simulink model "CM012A_FordT3McuCfg"  (R2013b)
settings: Solver=FixedStepDiscrete  SolverMode=SingleTasking  StartTime=0.0  StopTime=2  FixedStep=0.00005  RelTol=1e-3
values from neighbouring files (symbols this model uses):
  BATTVLTGSCAGFAC_ULS_F32 = DataDict.Constant    [CM012A_FordT3McuCfg_DataDict.m]
  BATTVLTGSWD1SCAGFAC_ULS_F32 = DataDict.Constant    [CM012A_FordT3McuCfg_DataDict.m]
  CHRGPMPDIAGSCAGFAC_ULS_F32 = DataDict.Constant    [CM012A_FordT3McuCfg_DataDict.m]
  MOTAG2MEAS_ECU1OFFS_MOTREV_F32 = DataDict.Constant    [CM012A_FordT3McuCfg_DataDict.m]
  MOTAG2MEAS_ECU2OFFS_MOTREV_F32 = DataDict.Constant    [CM012A_FordT3McuCfg_DataDict.m]
  PWRDISCNCTSWTDIAGSCAGFAC_ULS_F32 = DataDict.Constant    [CM012A_FordT3McuCfg_DataDict.m]
undefined symbols (not defined in the file or in its folder): HwAgSnsrTyp1, sigbuilder_block
libraries: CM012A_FordT3McuCfg_ModelLibrary x114, simulink x37, NxtrLim x34
(part 3 of 4)

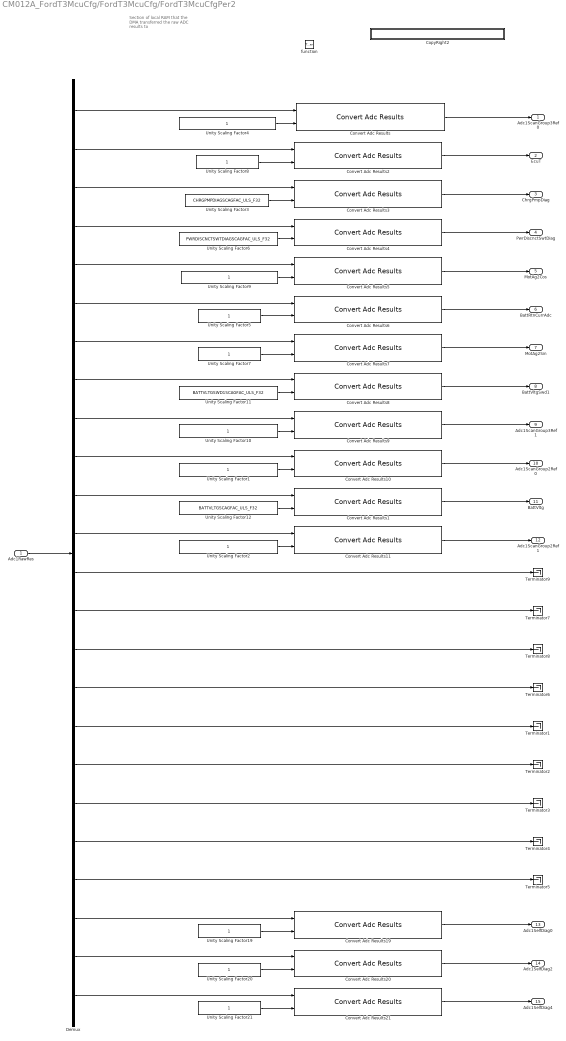
== system CM012A_FordT3McuCfg/FordT3McuCfg/FordT3McuCfgPer2 ==
  note: Section of local RAM that the
      | DMA transferred the raw
      | ADC results to
  Adc1RawRes : Inport
  function : TriggerPort  TriggerType=function-call
  Convert Adc Results{,9..11,19..21} (7 alike) : CM012A_FordT3McuCfg_ModelLibrary/Convert Adc Results
  Convert Adc Results1 : CM012A_FordT3McuCfg_ModelLibrary/Convert Adc Results  RequirementInfo="{'linktype_rmi_doors' '00016ba8 (/ESG Group/FDD Module Requirements/EA4 Specific/CM012A_FordT3McuCfg)' '#CM012A_185' 'true' 'REQ:  CM012A_185' '' } %GIDa_5e3dfbd3_0aa2_4a0d_bf3e_86a251f38de3"
  Convert Adc Results2 : CM012A_FordT3McuCfg_ModelLibrary/Convert Adc Results  RequirementInfo="{'linktype_rmi_doors' '00016ba8 (/ESG Group/FDD Module Requirements/EA4 Specific/CM012A_FordT3McuCfg)' '#CM012A_178' 'true' 'REQ:  CM012A_178' '' } %GIDa_a26960ee_7e00_4846_9982_291370be49c9"
  Convert Adc Results3 : CM012A_FordT3McuCfg_ModelLibrary/Convert Adc Results  RequirementInfo="{'linktype_rmi_doors' '00016ba8 (/ESG Group/FDD Module Requirements/EA4 Specific/CM012A_FordT3McuCfg)' '#CM012A_179' 'true' 'REQ:  CM012A_179' '' } %GIDa_a9d1aa2c_659d_4b57_940c_077b57984895"
  Convert Adc Results4 : CM012A_FordT3McuCfg_ModelLibrary/Convert Adc Results  RequirementInfo="{'linktype_rmi_doors' '00016ba8 (/ESG Group/FDD Module Requirements/EA4 Specific/CM012A_FordT3McuCfg)' '#CM012A_180' 'true' 'REQ:  CM012A_180' '' } %GIDa_849e543f_3e98_4047_be72_b68ed64419df"
  Convert Adc Results5 : CM012A_FordT3McuCfg_ModelLibrary/Convert Adc Results  RequirementInfo="{'linktype_rmi_doors' '00016ba8 (/ESG Group/FDD Module Requirements/EA4 Specific/CM012A_FordT3McuCfg)' '#CM012A_181' 'true' 'REQ:  CM012A_181' '' } %GIDa_b9fd61a2_c26d_490b_9ec2_e1953f6cec27"
  Convert Adc Results6 : CM012A_FordT3McuCfg_ModelLibrary/Convert Adc Results  RequirementInfo="{'linktype_rmi_doors' '00016ba8 (/ESG Group/FDD Module Requirements/EA4 Specific/CM012A_FordT3McuCfg)' '#CM012A_182' 'true' 'REQ:  CM012A_182' '' } %GIDa_1805e95d_a947_4975_b3f2_aa5b017a8660"
  Convert Adc Results7 : CM012A_FordT3McuCfg_ModelLibrary/Convert Adc Results  RequirementInfo="{'linktype_rmi_doors' '00016ba8 (/ESG Group/FDD Module Requirements/EA4 Specific/CM012A_FordT3McuCfg)' '#CM012A_183' 'true' 'REQ:  CM012A_183' '' } %GIDa_b0f2763e_6efc_4366_bdd2_7a7ad43f2cd5"
  Convert Adc Results8 : CM012A_FordT3McuCfg_ModelLibrary/Convert Adc Results  RequirementInfo="{'linktype_rmi_doors' '00016ba8 (/ESG Group/FDD Module Requirements/EA4 Specific/CM012A_FordT3McuCfg)' '#CM012A_184' 'true' 'REQ:  CM012A_184' '' } %GIDa_a85505f7_8cc5_414b_b13e_a958c65078c9"
  CopyRight2 : Subsystem  Description=|  mask(Copyright Information){none=on}
      | Copyright info block.                                               
      |                                                                     
      | Place copyright information at the top of every subsystem in design.
      mask prompts: none "No parameters"
      mask help: Place copyright information at the top of every subsystem in design.
      mask Display:
      | NxtrConf = 'Nexteer Confidential';
      | 
      | sys = bdroot; %handle for the current model ("system")
      | first = get_param(sys,'Created');
      | first = first(end-3:end);  %year is last four digits
      | 
      | last = get_param(sys,'LastModifiedDate');
      | if isempty(last)
      |     last = datestr(now,'yyyy');
      | else
      |     last = last(end-3:end);
      | end
      | 
      | if strcmp(first,last)
      |     fprintf('%s -- Copyright %s Nexteer',NxtrConf,first)
      | else
      |     fprintf('%s -- %s%s- %s Nexteer',NxtrConf,char(169),first,last)
      | end
  Demux : Demux  Outputs=24
  Terminator{1..9} (9 alike) : Terminator
  Unity Scaling Factor{1..2,4..5,7..10,19..21} (11 alike) : Constant  OutDataTypeStr=single
  Unity Scaling Factor11 : Constant  RequirementInfo="{'linktype_rmi_doors' '00016ba8 (/ESG Group/FDD Module Requirements/EA4 Specific/CM012A_FordT3McuCfg)' '#CM012A_184' 'true' 'REQ:  CM012A_184' '' } %GIDa_4557c3db_2e6a_4677_b8e3_15478f0550e6"  Value=BATTVLTGSWD1SCAGFAC_ULS_F32
  Unity Scaling Factor12 : Constant  RequirementInfo="{'linktype_rmi_doors' '00016ba8 (/ESG Group/FDD Module Requirements/EA4 Specific/CM012A_FordT3McuCfg)' '#CM012A_185' 'true' 'REQ:  CM012A_185' '' } %GIDa_1deb9cd3_1e38_4031_b7c6_d1408aef7916"  Value=BATTVLTGSCAGFAC_ULS_F32
  Unity Scaling Factor3 : Constant  RequirementInfo="{'linktype_rmi_doors' '00016ba8 (/ESG Group/FDD Module Requirements/EA4 Specific/CM012A_FordT3McuCfg)' '#CM012A_179' 'true' 'REQ:  CM012A_179' '' } %GIDa_de87164e_670f_496e_a314_697b1553e9fe"  Value=CHRGPMPDIAGSCAGFAC_ULS_F32
  Unity Scaling Factor6 : Constant  RequirementInfo="{'linktype_rmi_doors' '00016ba8 (/ESG Group/FDD Module Requirements/EA4 Specific/CM012A_FordT3McuCfg)' '#CM012A_180' 'true' 'REQ:  CM012A_180' '' } %GIDa_80971ee9_65a5_459a_87c3_3a33b74619be"  Value=PWRDISCNCTSWTDIAGSCAGFAC_ULS_F32
  Adc1ScanGroup3Ref0 : Outport
  EcuT : Outport  Port=2
  ChrgPmpDiag : Outport  Port=3
  PwrDiscnctSwtDiag : Outport  Port=4
  MotAg2Cos : Outport  Port=5
  BattRtnCurrAdc : Outport  Port=6
  MotAg2Sin : Outport  Port=7
  BattVltgSwd1 : Outport  Port=8
  Adc1ScanGroup3Ref1 : Outport  Port=9
  Adc1ScanGroup2Ref0 : Outport  Port=10
  BattVltg : Outport  Port=11
  Adc1ScanGroup2Ref1 : Outport  Port=12
  Adc1SelfDiag0 : Outport  Port=13
  Adc1SelfDiag2 : Outport  Port=14
  Adc1SelfDiag4 : Outport  Port=15
  wires:
  Adc1RawRes/1 -> Demux/1
  Demux/1 -> Convert Adc Results/1
  Unity Scaling Factor4/1 -> Convert Adc Results/2
  Convert Adc Results/1 -> Adc1ScanGroup3Ref0/1
  Demux/4 -> Convert Adc Results4/1
  Unity Scaling Factor3/1 -> Convert Adc Results3/2
  Demux/3 -> Convert Adc Results3/1
  Unity Scaling Factor8/1 -> Convert Adc Results2/2
  Demux/2 -> Convert Adc Results2/1
  Unity Scaling Factor6/1 -> Convert Adc Results4/2
  Demux/9 -> Convert Adc Results9/1
  Unity Scaling Factor11/1 -> Convert Adc Results8/2
  Demux/8 -> Convert Adc Results8/1
  Unity Scaling Factor7/1 -> Convert Adc Results7/2
  Demux/7 -> Convert Adc Results7/1
  Unity Scaling Factor5/1 -> Convert Adc Results6/2
  Demux/6 -> Convert Adc Results6/1
  Demux/5 -> Convert Adc Results5/1
  Unity Scaling Factor9/1 -> Convert Adc Results5/2
  Unity Scaling Factor10/1 -> Convert Adc Results9/2
  Convert Adc Results2/1 -> EcuT/1
  Convert Adc Results3/1 -> ChrgPmpDiag/1
  Convert Adc Results4/1 -> PwrDiscnctSwtDiag/1
  Convert Adc Results5/1 -> MotAg2Cos/1
  Convert Adc Results6/1 -> BattRtnCurrAdc/1
  Demux/10 -> Convert Adc Results10/1
  Unity Scaling Factor1/1 -> Convert Adc Results10/2
  Convert Adc Results7/1 -> MotAg2Sin/1
  Convert Adc Results8/1 -> BattVltgSwd1/1
  Convert Adc Results9/1 -> Adc1ScanGroup3Ref1/1
  Convert Adc Results10/1 -> Adc1ScanGroup2Ref0/1
  Unity Scaling Factor12/1 -> Convert Adc Results1/2
  Demux/11 -> Convert Adc Results1/1
  Convert Adc Results1/1 -> BattVltg/1
  Demux/17 -> Terminator1/1
  Demux/18 -> Terminator2/1
  Demux/19 -> Terminator3/1
  Demux/20 -> Terminator4/1
  Demux/21 -> Terminator5/1
  Unity Scaling Factor21/1 -> Convert Adc Results21/2
  Demux/24 -> Convert Adc Results21/1
  Unity Scaling Factor20/1 -> Convert Adc Results20/2
  Demux/23 -> Convert Adc Results20/1
  Unity Scaling Factor19/1 -> Convert Adc Results19/2
  Demux/22 -> Convert Adc Results19/1
  Demux/12 -> Convert Adc Results11/1
  Unity Scaling Factor2/1 -> Convert Adc Results11/2
  Demux/16 -> Terminator6/1
  Demux/14 -> Terminator7/1
  Demux/15 -> Terminator8/1
  Demux/13 -> Terminator9/1
  Convert Adc Results11/1 -> Adc1ScanGroup2Ref1/1
  Convert Adc Results20/1 -> Adc1SelfDiag2/1
  Convert Adc Results19/1 -> Adc1SelfDiag0/1
  Convert Adc Results21/1 -> Adc1SelfDiag4/1

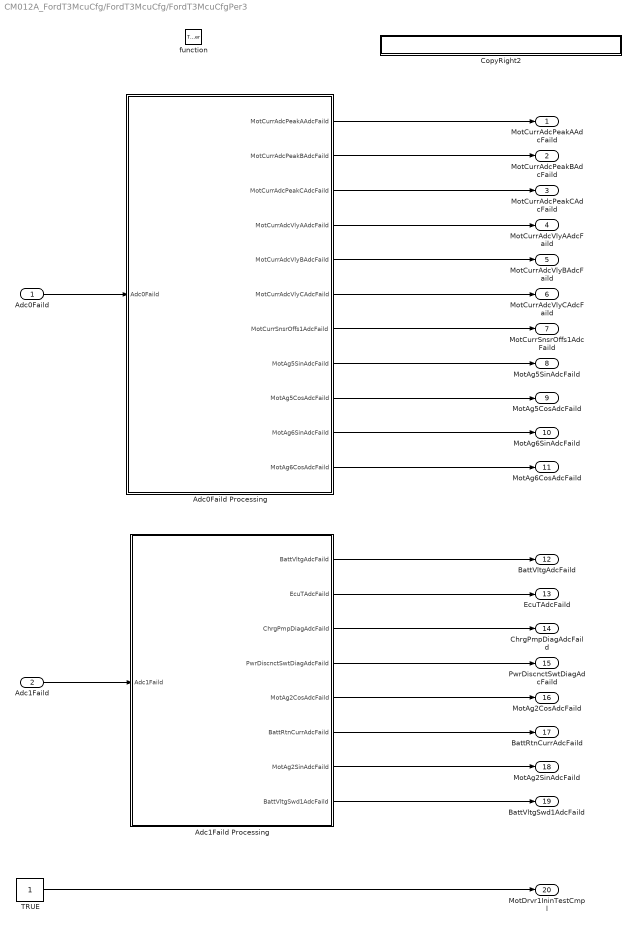
== system CM012A_FordT3McuCfg/FordT3McuCfg/FordT3McuCfgPer3 ==
  Adc0Faild : Inport
  Adc1Faild : Inport  Port=2
  function : TriggerPort  TriggerType=function-call
  Adc0Faild Processing : Subsystem  TreatAsAtomicUnit=on
  Adc1Faild Processing : Subsystem  TreatAsAtomicUnit=on
  CopyRight2 : Subsystem  Description=|  mask(Copyright Information){none=on}
      | Copyright info block.                                               
      |                                                                     
      | Place copyright information at the top of every subsystem in design.
      mask prompts: none "No parameters"
      mask help: Place copyright information at the top of every subsystem in design.
      mask Display:
      | NxtrConf = 'Nexteer Confidential';
      | 
      | sys = bdroot; %handle for the current model ("system")
      | first = get_param(sys,'Created');
      | first = first(end-3:end);  %year is last four digits
      | 
      | last = get_param(sys,'LastModifiedDate');
      | if isempty(last)
      |     last = datestr(now,'yyyy');
      | else
      |     last = last(end-3:end);
      | end
      | 
      | if strcmp(first,last)
      |     fprintf('%s -- Copyright %s Nexteer',NxtrConf,first)
      | else
      |     fprintf('%s -- %s%s- %s Nexteer',NxtrConf,char(169),first,last)
      | end
  TRUE : Constant
  MotCurrAdcPeakAAdcFaild : Outport
  MotCurrAdcPeakBAdcFaild : Outport  Port=2
  MotCurrAdcPeakCAdcFaild : Outport  Port=3
  MotCurrAdcVlyAAdcFaild : Outport  Port=4
  MotCurrAdcVlyBAdcFaild : Outport  Port=5
  MotCurrAdcVlyCAdcFaild : Outport  Port=6
  MotCurrSnsrOffs1AdcFaild : Outport  Port=7
  MotAg5SinAdcFaild : Outport  Port=8
  MotAg5CosAdcFaild : Outport  Port=9
  MotAg6SinAdcFaild : Outport  Port=10
  MotAg6CosAdcFaild : Outport  Port=11
  BattVltgAdcFaild : Outport  Port=12
  EcuTAdcFaild : Outport  Port=13
  ChrgPmpDiagAdcFaild : Outport  Port=14
  PwrDiscnctSwtDiagAdcFaild : Outport  Port=15
  MotAg2CosAdcFaild : Outport  Port=16
  BattRtnCurrAdcFaild : Outport  Port=17
  MotAg2SinAdcFaild : Outport  Port=18
  BattVltgSwd1AdcFaild : Outport  Port=19
  MotDrvr1IninTestCmpl : Outport  Port=20
  wires:
  Adc0Faild/1 -> Adc0Faild Processing/1(Adc0Faild)
  Adc1Faild/1 -> Adc1Faild Processing/1(Adc1Faild)
  Adc0Faild Processing/11(MotAg6CosAdcFaild) -> MotAg6CosAdcFaild/1
  Adc0Faild Processing/10(MotAg6SinAdcFaild) -> MotAg6SinAdcFaild/1
  Adc0Faild Processing/9(MotAg5CosAdcFaild) -> MotAg5CosAdcFaild/1
  Adc0Faild Processing/8(MotAg5SinAdcFaild) -> MotAg5SinAdcFaild/1
  Adc0Faild Processing/7(MotCurrSnsrOffs1AdcFaild) -> MotCurrSnsrOffs1AdcFaild/1
  Adc0Faild Processing/6(MotCurrAdcVlyCAdcFaild) -> MotCurrAdcVlyCAdcFaild/1
  Adc0Faild Processing/5(MotCurrAdcVlyBAdcFaild) -> MotCurrAdcVlyBAdcFaild/1
  Adc0Faild Processing/4(MotCurrAdcVlyAAdcFaild) -> MotCurrAdcVlyAAdcFaild/1
  Adc0Faild Processing/3(MotCurrAdcPeakCAdcFaild) -> MotCurrAdcPeakCAdcFaild/1
  Adc0Faild Processing/2(MotCurrAdcPeakBAdcFaild) -> MotCurrAdcPeakBAdcFaild/1
  Adc0Faild Processing/1(MotCurrAdcPeakAAdcFaild) -> MotCurrAdcPeakAAdcFaild/1
  Adc1Faild Processing/1(BattVltgAdcFaild) -> BattVltgAdcFaild/1
  Adc1Faild Processing/2(EcuTAdcFaild) -> EcuTAdcFaild/1
  Adc1Faild Processing/3(ChrgPmpDiagAdcFaild) -> ChrgPmpDiagAdcFaild/1
  Adc1Faild Processing/4(PwrDiscnctSwtDiagAdcFaild) -> PwrDiscnctSwtDiagAdcFaild/1
  Adc1Faild Processing/5(MotAg2CosAdcFaild) -> MotAg2CosAdcFaild/1
  Adc1Faild Processing/6(BattRtnCurrAdcFaild) -> BattRtnCurrAdcFaild/1
  Adc1Faild Processing/7(MotAg2SinAdcFaild) -> MotAg2SinAdcFaild/1
  Adc1Faild Processing/8(BattVltgSwd1AdcFaild) -> BattVltgSwd1AdcFaild/1
  TRUE/1 -> MotDrvr1IninTestCmpl/1

== system CM012A_FordT3McuCfg/FordT3McuCfg/FordT3McuCfgInit1/CopyRight2 ==

== system CM012A_FordT3McuCfg/FordT3McuCfg/FordT3McuCfgInit1/Register Initialization ==
  note: FordT3McuCfg Configuration
      | Power Down Mode Register Initialization, Have to be part of Start-up sequence
      | Run this before all other init functions.
      |
      | CM012A_FordT3McuCfg_PowerDownModeRegisterConfiguration.xlsm
  CopyRight2 : Subsystem  Description=|  mask(Copyright Information){none=on}
      | Copyright info block.                                               
      |                                                                     
      | Place copyright information at the top of every subsystem in design.
      mask prompts: none "No parameters"
      mask help: Place copyright information at the top of every subsystem in design.
      mask Display:
      | NxtrConf = 'Nexteer Confidential';
      | 
      | sys = bdroot; %handle for the current model ("system")
      | first = get_param(sys,'Created');
      | first = first(end-3:end);  %year is last four digits
      | 
      | last = get_param(sys,'LastModifiedDate');
      | if isempty(last)
      |     last = datestr(now,'yyyy');
      | else
      |     last = last(end-3:end);
      | end
      | 
      | if strcmp(first,last)
      |     fprintf('%s -- Copyright %s Nexteer',NxtrConf,first)
      | else
      |     fprintf('%s -- %s%s- %s Nexteer',NxtrConf,char(169),first,last)
      | end

== system CM012A_FordT3McuCfg/FordT3McuCfg/FordT3McuCfgInit2/CopyRight2 ==

== system CM012A_FordT3McuCfg/FordT3McuCfg/FordT3McuCfgInit2/Register Initialization ==
  note: FordT3McuCfg Configuration
      | Initialize the PIC registers from the following sources in the order listed:
      |
      |
      | 1. Run Adcf0CfgAndUseInit1 - this means to run the AdcCfgInit function first before this init function, there is no client or server call
      | 2  Run Adcf1CfgAndUseInit1 - this means to run the AdcCfgInit function first before this init function, there is no client or server call
      | 3. CM012A_FordT3McuCfg_PICRegisterConfiguration.xlsm
      |     Order by row
  CopyRight2 : Subsystem  Description=|  mask(Copyright Information){none=on}
      | Copyright info block.                                               
      |                                                                     
      | Place copyright information at the top of every subsystem in design.
      mask prompts: none "No parameters"
      mask help: Place copyright information at the top of every subsystem in design.
      mask Display:
      | NxtrConf = 'Nexteer Confidential';
      | 
      | sys = bdroot; %handle for the current model ("system")
      | first = get_param(sys,'Created');
      | first = first(end-3:end);  %year is last four digits
      | 
      | last = get_param(sys,'LastModifiedDate');
      | if isempty(last)
      |     last = datestr(now,'yyyy');
      | else
      |     last = last(end-3:end);
      | end
      | 
      | if strcmp(first,last)
      |     fprintf('%s -- Copyright %s Nexteer',NxtrConf,first)
      | else
      |     fprintf('%s -- %s%s- %s Nexteer',NxtrConf,char(169),first,last)
      | end

== system CM012A_FordT3McuCfg/FordT3McuCfg/FordT3McuCfgInit3/CopyRight2 ==

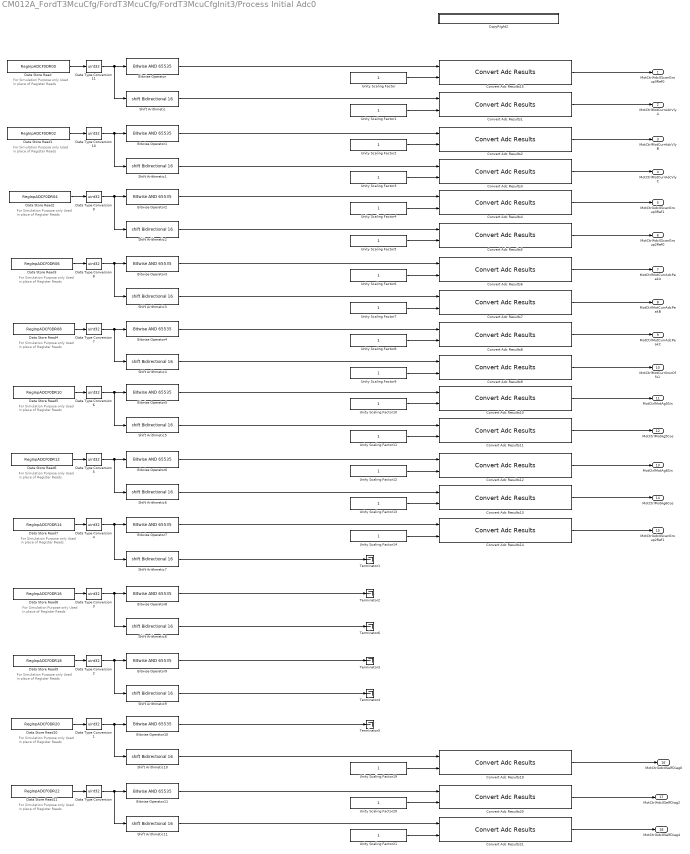
== system CM012A_FordT3McuCfg/FordT3McuCfg/FordT3McuCfgInit3/Process Initial Adc0 ==
  note: For Simulation Purpose only
      | Used in place of Register Reads
  note: For Simulation Purpose only
      | Used in place of Register Reads
  note: For Simulation Purpose only
      | Used in place of Register Reads
  note: For Simulation Purpose only
      | Used in place of Register Reads
  note: For Simulation Purpose only
      | Used in place of Register Reads
  note: For Simulation Purpose only
      | Used in place of Register Reads
  note: For Simulation Purpose only
      | Used in place of Register Reads
  note: For Simulation Purpose only
      | Used in place of Register Reads
  note: For Simulation Purpose only
      | Used in place of Register Reads
  note: For Simulation Purpose only
      | Used in place of Register Reads
  note: For Simulation Purpose only
      | Used in place of Register Reads
  note: For Simulation Purpose only
      | Used in place of Register Reads
  Bitwise Operator{,1..11} (12 alike) : simulink/Logic and Bit Operations/Bitwise Operator  logicop=AND  UseBitMask=on  BitMask=65535  BitMaskRealWorld=Stored Integer
  Convert Adc Results1 : CM012A_FordT3McuCfg_ModelLibrary/Convert Adc Results  RequirementInfo="{'linktype_rmi_doors' '00016ba8 (/ESG Group/FDD Module Requirements/EA4 Specific/CM012A_FordT3McuCfg)' '#CM012A_38' 'true' 'REQ:  CM012A_38' '' } %GIDa_a8dbc091_4b9a_46c5_99e0_ef4d9fb26bcb"
  Convert Adc Results10 : CM012A_FordT3McuCfg_ModelLibrary/Convert Adc Results  RequirementInfo="{'linktype_rmi_doors' '00016ba8 (/ESG Group/FDD Module Requirements/EA4 Specific/CM012A_FordT3McuCfg)' '#CM012A_174' 'true' 'REQ:  CM012A_174' '' } %GIDa_c713d23c_035e_47cc_b29e_17f4bade944f"
  Convert Adc Results11 : CM012A_FordT3McuCfg_ModelLibrary/Convert Adc Results  RequirementInfo="{'linktype_rmi_doors' '00016ba8 (/ESG Group/FDD Module Requirements/EA4 Specific/CM012A_FordT3McuCfg)' '#CM012A_175' 'true' 'REQ:  CM012A_175' '' } %GIDa_44f2e841_73df_47e4_be7b_03eceb97c083"
  Convert Adc Results12 : CM012A_FordT3McuCfg_ModelLibrary/Convert Adc Results  RequirementInfo="{'linktype_rmi_doors' '00016ba8 (/ESG Group/FDD Module Requirements/EA4 Specific/CM012A_FordT3McuCfg)' '#CM012A_176' 'true' 'REQ:  CM012A_176' '' } %GIDa_3df3459b_db95_4ccb_9a4e_0d74195d6582"
  Convert Adc Results13 : CM012A_FordT3McuCfg_ModelLibrary/Convert Adc Results  RequirementInfo="{'linktype_rmi_doors' '00016ba8 (/ESG Group/FDD Module Requirements/EA4 Specific/CM012A_FordT3McuCfg)' '#CM012A_177' 'true' 'REQ:  CM012A_177' '' } %GIDa_c37cf5b7_6415_4e96_9950_9119ecd6b065"
  Convert Adc Results{4..5,14..15,19..21} (7 alike) : CM012A_FordT3McuCfg_ModelLibrary/Convert Adc Results
  Convert Adc Results2 : CM012A_FordT3McuCfg_ModelLibrary/Convert Adc Results  RequirementInfo="{'linktype_rmi_doors' '00016ba8 (/ESG Group/FDD Module Requirements/EA4 Specific/CM012A_FordT3McuCfg)' '#CM012A_122' 'true' 'REQ:  CM012A_122' '' } %GIDa_c712f731_3a74_4ffe_b868_79dfb504de9e"
  Convert Adc Results3 : CM012A_FordT3McuCfg_ModelLibrary/Convert Adc Results  RequirementInfo="{'linktype_rmi_doors' '00016ba8 (/ESG Group/FDD Module Requirements/EA4 Specific/CM012A_FordT3McuCfg)' '#CM012A_126' 'true' 'REQ:  CM012A_126' '' } %GIDa_aefb9bef_da5f_4ab0_b36f_ae0b99865ccd"
  Convert Adc Results6 : CM012A_FordT3McuCfg_ModelLibrary/Convert Adc Results  RequirementInfo="{'linktype_rmi_doors' '00016ba8 (/ESG Group/FDD Module Requirements/EA4 Specific/CM012A_FordT3McuCfg)' '#CM012A_170' 'true' 'REQ:  CM012A_170' '' } %GIDa_f8a267c1_80d9_4509_ac0d_306d4e9a72ee"
  Convert Adc Results7 : CM012A_FordT3McuCfg_ModelLibrary/Convert Adc Results  RequirementInfo="{'linktype_rmi_doors' '00016ba8 (/ESG Group/FDD Module Requirements/EA4 Specific/CM012A_FordT3McuCfg)' '#CM012A_171' 'true' 'REQ:  CM012A_171' '' } %GIDa_9fa57759_dca7_4a57_9172_23edc1096740"
  Convert Adc Results8 : CM012A_FordT3McuCfg_ModelLibrary/Convert Adc Results  RequirementInfo="{'linktype_rmi_doors' '00016ba8 (/ESG Group/FDD Module Requirements/EA4 Specific/CM012A_FordT3McuCfg)' '#CM012A_172' 'true' 'REQ:  CM012A_172' '' } %GIDa_ee12c5b1_007c_4e26_b45a_3a2444b6883e"
  Convert Adc Results9 : CM012A_FordT3McuCfg_ModelLibrary/Convert Adc Results  RequirementInfo="{'linktype_rmi_doors' '00016ba8 (/ESG Group/FDD Module Requirements/EA4 Specific/CM012A_FordT3McuCfg)' '#CM012A_173' 'true' 'REQ:  CM012A_173' '' } %GIDa_656ea52f_0acd_4f6c_b662_ac0e1e909578"
  CopyRight2 : Subsystem  Description=|  mask(Copyright Information){none=on}
      | Copyright info block.                                               
      |                                                                     
      | Place copyright information at the top of every subsystem in design.
      mask prompts: none "No parameters"
      mask help: Place copyright information at the top of every subsystem in design.
      mask Display:
      | NxtrConf = 'Nexteer Confidential';
      | 
      | sys = bdroot; %handle for the current model ("system")
      | first = get_param(sys,'Created');
      | first = first(end-3:end);  %year is last four digits
      | 
      | last = get_param(sys,'LastModifiedDate');
      | if isempty(last)
      |     last = datestr(now,'yyyy');
      | else
      |     last = last(end-3:end);
      | end
      | 
      | if strcmp(first,last)
      |     fprintf('%s -- Copyright %s Nexteer',NxtrConf,first)
      | else
      |     fprintf('%s -- %s%s- %s Nexteer',NxtrConf,char(169),first,last)
      | end
  Data Store Read : DataStoreRead  DataStoreName=RegInpADCF0DR00
  Data Store Read1 : DataStoreRead  DataStoreName=RegInpADCF0DR02
  Data Store Read10 : DataStoreRead  DataStoreName=RegInpADCF0DR20
  Data Store Read11 : DataStoreRead  DataStoreName=RegInpADCF0DR22
  Data Store Read2 : DataStoreRead  DataStoreName=RegInpADCF0DR04
  Data Store Read3 : DataStoreRead  DataStoreName=RegInpADCF0DR06
  Data Store Read4 : DataStoreRead  DataStoreName=RegInpADCF0DR08
  Data Store Read5 : DataStoreRead  DataStoreName=RegInpADCF0DR10
  Data Store Read6 : DataStoreRead  DataStoreName=RegInpADCF0DR12
  Data Store Read7 : DataStoreRead  DataStoreName=RegInpADCF0DR14
  Data Store Read8 : DataStoreRead  DataStoreName=RegInpADCF0DR16
  Data Store Read9 : DataStoreRead  DataStoreName=RegInpADCF0DR18
  Data Type Conversion{,1..11} (12 alike) : DataTypeConversion  OutDataTypeStr=uint32
  Shift Arithmetic{,1..11} (12 alike) : ArithShift  BitShiftNumber=16
  Terminator{1..6} (6 alike) : Terminator
  Unity Scaling Factor{,1..14,19..21} (18 alike) : Constant  OutDataTypeStr=single
  MotCtrlAdc0ScanGroup3Ref0 : Outport
  MotCtrlMotCurrAdcVlyA : Outport  Port=2
  MotCtrlMotCurrAdcVlyB : Outport  Port=3
  MotCtrlMotCurrAdcVlyC : Outport  Port=4
  MotCtrlAdc0ScanGroup3Ref1 : Outport  Port=5
  MotCtrlAdc0ScanGroup2Ref0 : Outport  Port=6
  MotCtrlMotCurrAdcPeakA : Outport  Port=7
  MotCtrlMotCurrAdcPeakB : Outport  Port=8
  MotCtrlMotCurrAdcPeakC : Outport  Port=9
  MotCtrlMotCurrSnsrOffs1 : Outport  Port=10
  MotCtrlMotAg5Sin : Outport  Port=11
  MotCtrlMotAg5Cos : Outport  Port=12
  MotCtrlMotAg6Sin : Outport  Port=13
  MotCtrlMotAg6Cos : Outport  Port=14
  MotCtrlAdc0ScanGroup2Ref1 : Outport  Port=15
  MotCtrlAdc0SelfDiag0 : Outport  Port=16
  MotCtrlAdc0SelfDiag2 : Outport  Port=17
  MotCtrlAdc0SelfDiag4 : Outport  Port=18
  wires:
  Bitwise Operator/1 -> Convert Adc Results15/1
  Unity Scaling Factor/1 -> Convert Adc Results15/2
  Shift Arithmetic/1 -> Convert Adc Results1/1
  Unity Scaling Factor1/1 -> Convert Adc Results1/2
  Unity Scaling Factor2/1 -> Convert Adc Results2/2
  Unity Scaling Factor3/1 -> Convert Adc Results3/2
  Unity Scaling Factor4/1 -> Convert Adc Results4/2
  Unity Scaling Factor5/1 -> Convert Adc Results5/2
  Unity Scaling Factor6/1 -> Convert Adc Results6/2
  Unity Scaling Factor7/1 -> Convert Adc Results7/2
  Unity Scaling Factor8/1 -> Convert Adc Results8/2
  Unity Scaling Factor19/1 -> Convert Adc Results19/2
  Unity Scaling Factor20/1 -> Convert Adc Results20/2
  Unity Scaling Factor21/1 -> Convert Adc Results21/2
  Bitwise Operator1/1 -> Convert Adc Results2/1
  Shift Arithmetic1/1 -> Convert Adc Results3/1
  Shift Arithmetic11/1 -> Convert Adc Results21/1
  Bitwise Operator11/1 -> Convert Adc Results20/1
  Shift Arithmetic10/1 -> Convert Adc Results19/1
  Bitwise Operator10/1 -> Terminator5/1
  Bitwise Operator9/1 -> Terminator3/1
  Shift Arithmetic9/1 -> Terminator4/1
  Bitwise Operator4/1 -> Convert Adc Results8/1
  Bitwise Operator3/1 -> Convert Adc Results6/1
  Shift Arithmetic3/1 -> Convert Adc Results7/1
  Bitwise Operator2/1 -> Convert Adc Results4/1
  Shift Arithmetic2/1 -> Convert Adc Results5/1
  Unity Scaling Factor9/1 -> Convert Adc Results9/2
  Unity Scaling Factor10/1 -> Convert Adc Results10/2
  Unity Scaling Factor11/1 -> Convert Adc Results11/2
  Unity Scaling Factor12/1 -> Convert Adc Results12/2
  Unity Scaling Factor13/1 -> Convert Adc Results13/2
  Unity Scaling Factor14/1 -> Convert Adc Results14/2
  Shift Arithmetic4/1 -> Convert Adc Results9/1
  Bitwise Operator7/1 -> Convert Adc Results14/1
  Bitwise Operator6/1 -> Convert Adc Results12/1
  Shift Arithmetic6/1 -> Convert Adc Results13/1
  Bitwise Operator5/1 -> Convert Adc Results10/1
  Shift Arithmetic5/1 -> Convert Adc Results11/1
  Shift Arithmetic8/1 -> Terminator6/1
  Shift Arithmetic7/1 -> Terminator1/1
  Bitwise Operator8/1 -> Terminator2/1
  Data Type Conversion/1 -> Bitwise Operator11/1, Shift Arithmetic11/1
  Data Type Conversion1/1 -> Bitwise Operator10/1, Shift Arithmetic10/1
  Data Type Conversion2/1 -> Bitwise Operator9/1, Shift Arithmetic9/1
  Data Type Conversion3/1 -> Bitwise Operator8/1, Shift Arithmetic8/1
  Data Type Conversion4/1 -> Bitwise Operator7/1, Shift Arithmetic7/1
  Data Type Conversion5/1 -> Bitwise Operator6/1, Shift Arithmetic6/1
  Data Type Conversion6/1 -> Bitwise Operator5/1, Shift Arithmetic5/1
  Data Type Conversion7/1 -> Bitwise Operator4/1, Shift Arithmetic4/1
  Data Type Conversion8/1 -> Bitwise Operator3/1, Shift Arithmetic3/1
  Data Type Conversion9/1 -> Bitwise Operator2/1, Shift Arithmetic2/1
  Data Type Conversion10/1 -> Bitwise Operator1/1, Shift Arithmetic1/1
  Data Type Conversion11/1 -> Bitwise Operator/1, Shift Arithmetic/1
  Data Store Read/1 -> Data Type Conversion11/1
  Data Store Read2/1 -> Data Type Conversion9/1
  Data Store Read3/1 -> Data Type Conversion8/1
  Data Store Read4/1 -> Data Type Conversion7/1
  Data Store Read5/1 -> Data Type Conversion6/1
  Data Store Read6/1 -> Data Type Conversion5/1
  Data Store Read7/1 -> Data Type Conversion4/1
  Data Store Read8/1 -> Data Type Conversion3/1
  Data Store Read9/1 -> Data Type Conversion2/1
  Data Store Read10/1 -> Data Type Conversion1/1
  Data Store Read11/1 -> Data Type Conversion/1
  Data Store Read1/1 -> Data Type Conversion10/1
  Convert Adc Results15/1 -> MotCtrlAdc0ScanGroup3Ref0/1
  Convert Adc Results1/1 -> MotCtrlMotCurrAdcVlyA/1
  Convert Adc Results2/1 -> MotCtrlMotCurrAdcVlyB/1
  Convert Adc Results3/1 -> MotCtrlMotCurrAdcVlyC/1
  Convert Adc Results4/1 -> MotCtrlAdc0ScanGroup3Ref1/1
  Convert Adc Results5/1 -> MotCtrlAdc0ScanGroup2Ref0/1
  Convert Adc Results6/1 -> MotCtrlMotCurrAdcPeakA/1
  Convert Adc Results7/1 -> MotCtrlMotCurrAdcPeakB/1
  Convert Adc Results8/1 -> MotCtrlMotCurrAdcPeakC/1
  Convert Adc Results9/1 -> MotCtrlMotCurrSnsrOffs1/1
  Convert Adc Results10/1 -> MotCtrlMotAg5Sin/1
  Convert Adc Results11/1 -> MotCtrlMotAg5Cos/1
  Convert Adc Results13/1 -> MotCtrlMotAg6Cos/1
  Convert Adc Results12/1 -> MotCtrlMotAg6Sin/1
  Convert Adc Results14/1 -> MotCtrlAdc0ScanGroup2Ref1/1
  Convert Adc Results19/1 -> MotCtrlAdc0SelfDiag0/1
  Convert Adc Results20/1 -> MotCtrlAdc0SelfDiag2/1
  Convert Adc Results21/1 -> MotCtrlAdc0SelfDiag4/1

== system CM012A_FordT3McuCfg/FordT3McuCfg/FordT3McuCfgInit3/Wait for ADC Conversion to Complete ==
  note: Use the following client calls to perform a 25uSec wait.
  CopyRight2 : Subsystem  Description=|  mask(Copyright Information){none=on}
      | Copyright info block.                                               
      |                                                                     
      | Place copyright information at the top of every subsystem in design.
      mask prompts: none "No parameters"
      mask help: Place copyright information at the top of every subsystem in design.
      mask Display:
      | NxtrConf = 'Nexteer Confidential';
      | 
      | sys = bdroot; %handle for the current model ("system")
      | first = get_param(sys,'Created');
      | first = first(end-3:end);  %year is last four digits
      | 
      | last = get_param(sys,'LastModifiedDate');
      | if isempty(last)
      |     last = datestr(now,'yyyy');
      | else
      |     last = last(end-3:end);
      | end
      | 
      | if strcmp(first,last)
      |     fprintf('%s -- Copyright %s Nexteer',NxtrConf,first)
      | else
      |     fprintf('%s -- %s%s- %s Nexteer',NxtrConf,char(169),first,last)
      | end
  GetRefTmr1MicroSec32bit : Subsystem  RequirementInfo="{'linktype_rmi_doors' '00016ba8 (/ESG Group/FDD Module Requirements/EA4 Specific/CM012A_FordT3McuCfg)' '#CM012A_115' 'true' 'REQ:  CM012A_115' '' } %GIDa_9f89a498_44a7_4edb_af20_9272e53781e3"  TreatAsAtomicUnit=on
  GetTiSpan1MicroSec32bit : Subsystem  RequirementInfo="{'linktype_rmi_doors' '00016ba8 (/ESG Group/FDD Module Requirements/EA4 Specific/CM012A_FordT3McuCfg)' '#CM012A_116' 'true' 'REQ:  CM012A_116' '' } %GIDa_ce85625c_3f35_4a51_b950_dd406ee43e06"  TreatAsAtomicUnit=on
  Ground : Ground
  Terminator : Terminator
  Terminator1 : Terminator
  wires:
  GetRefTmr1MicroSec32bit/1(RefTmr) -> Terminator/1
  GetTiSpan1MicroSec32bit/1(TiSpan) -> Terminator1/1
  Ground/1 -> GetTiSpan1MicroSec32bit/1(RefTmr)

== system CM012A_FordT3McuCfg/FordT3McuCfg/FordT3McuCfgInit4/CopyRight2 ==

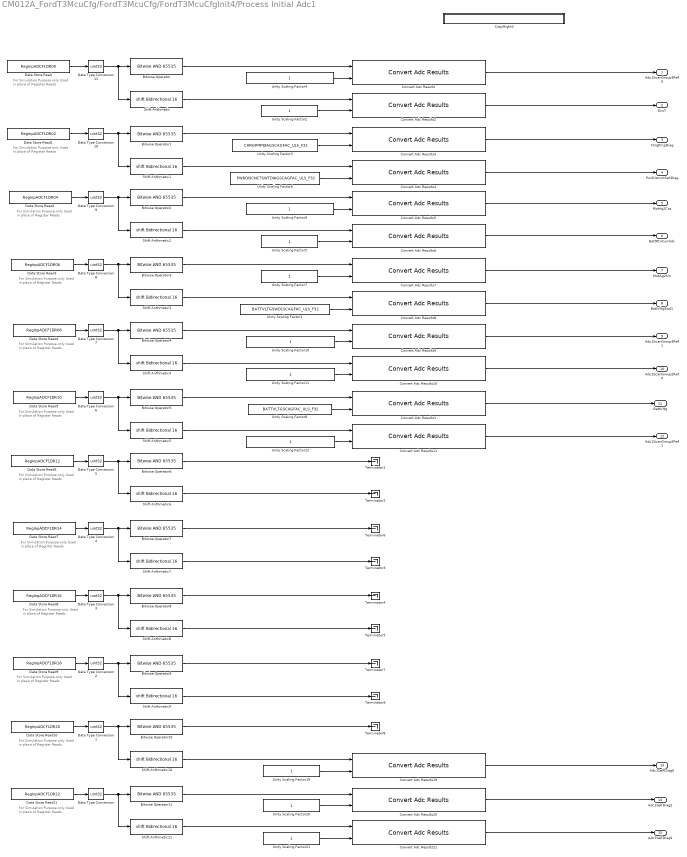
== system CM012A_FordT3McuCfg/FordT3McuCfg/FordT3McuCfgInit4/Process Initial Adc1 ==
  note: For Simulation Purpose only
      | Used in place of Register Reads
  note: For Simulation Purpose only
      | Used in place of Register Reads
  note: For Simulation Purpose only
      | Used in place of Register Reads
  note: For Simulation Purpose only
      | Used in place of Register Reads
  note: For Simulation Purpose only
      | Used in place of Register Reads
  note: For Simulation Purpose only
      | Used in place of Register Reads
  note: For Simulation Purpose only
      | Used in place of Register Reads
  note: For Simulation Purpose only
      | Used in place of Register Reads
  note: For Simulation Purpose only
      | Used in place of Register Reads
  note: For Simulation Purpose only
      | Used in place of Register Reads
  note: For Simulation Purpose only
      | Used in place of Register Reads
  note: For Simulation Purpose only
      | Used in place of Register Reads
  Bitwise Operator{,1..11} (12 alike) : simulink/Logic and Bit Operations/Bitwise Operator  logicop=AND  UseBitMask=on  BitMask=65535  BitMaskRealWorld=Stored Integer
  Convert Adc Results{,9..11,19..21} (7 alike) : CM012A_FordT3McuCfg_ModelLibrary/Convert Adc Results
  Convert Adc Results1 : CM012A_FordT3McuCfg_ModelLibrary/Convert Adc Results  RequirementInfo="{'linktype_rmi_doors' '00016ba8 (/ESG Group/FDD Module Requirements/EA4 Specific/CM012A_FordT3McuCfg)' '#CM012A_185' 'true' 'REQ:  CM012A_185' '' } %GIDa_4d834612_c0b7_4a13_9197_5805f5f3e4a8"
  Convert Adc Results2 : CM012A_FordT3McuCfg_ModelLibrary/Convert Adc Results  RequirementInfo="{'linktype_rmi_doors' '00016ba8 (/ESG Group/FDD Module Requirements/EA4 Specific/CM012A_FordT3McuCfg)' '#CM012A_178' 'true' 'REQ:  CM012A_178' '' } %GIDa_1348d1eb_e603_49ac_8bdf_adfe30d2b6cf"
  Convert Adc Results3 : CM012A_FordT3McuCfg_ModelLibrary/Convert Adc Results  RequirementInfo="{'linktype_rmi_doors' '00016ba8 (/ESG Group/FDD Module Requirements/EA4 Specific/CM012A_FordT3McuCfg)' '#CM012A_179' 'true' 'REQ:  CM012A_179' '' } %GIDa_f34fcb55_af62_4913_b97c_9ccfd1fd6802"
  Convert Adc Results4 : CM012A_FordT3McuCfg_ModelLibrary/Convert Adc Results  RequirementInfo="{'linktype_rmi_doors' '00016ba8 (/ESG Group/FDD Module Requirements/EA4 Specific/CM012A_FordT3McuCfg)' '#CM012A_180' 'true' 'REQ:  CM012A_180' '' } %GIDa_65ea6f30_a3b5_4550_a80a_a6709e47edd5"
  Convert Adc Results5 : CM012A_FordT3McuCfg_ModelLibrary/Convert Adc Results  RequirementInfo="{'linktype_rmi_doors' '00016ba8 (/ESG Group/FDD Module Requirements/EA4 Specific/CM012A_FordT3McuCfg)' '#CM012A_181' 'true' 'REQ:  CM012A_181' '' } %GIDa_79a03b87_5461_4058_81ce_16ee2dcf53c2"
  Convert Adc Results6 : CM012A_FordT3McuCfg_ModelLibrary/Convert Adc Results  RequirementInfo="{'linktype_rmi_doors' '00016ba8 (/ESG Group/FDD Module Requirements/EA4 Specific/CM012A_FordT3McuCfg)' '#CM012A_182' 'true' 'REQ:  CM012A_182' '' } %GIDa_2330a655_4975_4937_9bb7_1118e9074fb7"
  Convert Adc Results7 : CM012A_FordT3McuCfg_ModelLibrary/Convert Adc Results  RequirementInfo="{'linktype_rmi_doors' '00016ba8 (/ESG Group/FDD Module Requirements/EA4 Specific/CM012A_FordT3McuCfg)' '#CM012A_183' 'true' 'REQ:  CM012A_183' '' } %GIDa_b5355b0e_838c_4331_88c8_b1d62810f1f0"
  Convert Adc Results8 : CM012A_FordT3McuCfg_ModelLibrary/Convert Adc Results  RequirementInfo="{'linktype_rmi_doors' '00016ba8 (/ESG Group/FDD Module Requirements/EA4 Specific/CM012A_FordT3McuCfg)' '#CM012A_184' 'true' 'REQ:  CM012A_184' '' } %GIDa_fbdd6cd6_4808_4987_9cdf_ffe8ea3c7dd4"
  CopyRight2 : Subsystem  Description=|  mask(Copyright Information){none=on}
      | Copyright info block.                                               
      |                                                                     
      | Place copyright information at the top of every subsystem in design.
      mask prompts: none "No parameters"
      mask help: Place copyright information at the top of every subsystem in design.
      mask Display:
      | NxtrConf = 'Nexteer Confidential';
      | 
      | sys = bdroot; %handle for the current model ("system")
      | first = get_param(sys,'Created');
      | first = first(end-3:end);  %year is last four digits
      | 
      | last = get_param(sys,'LastModifiedDate');
      | if isempty(last)
      |     last = datestr(now,'yyyy');
      | else
      |     last = last(end-3:end);
      | end
      | 
      | if strcmp(first,last)
      |     fprintf('%s -- Copyright %s Nexteer',NxtrConf,first)
      | else
      |     fprintf('%s -- %s%s- %s Nexteer',NxtrConf,char(169),first,last)
      | end
  Data Store Read : DataStoreRead  DataStoreName=RegInpADCF1DR00
  Data Store Read1 : DataStoreRead  DataStoreName=RegInpADCF1DR02
  Data Store Read10 : DataStoreRead  DataStoreName=RegInpADCF1DR20
  Data Store Read11 : DataStoreRead  DataStoreName=RegInpADCF1DR22
  Data Store Read2 : DataStoreRead  DataStoreName=RegInpADCF1DR04
  Data Store Read3 : DataStoreRead  DataStoreName=RegInpADCF1DR06
  Data Store Read4 : DataStoreRead  DataStoreName=RegInpADCF1DR08
  Data Store Read5 : DataStoreRead  DataStoreName=RegInpADCF1DR10
  Data Store Read6 : DataStoreRead  DataStoreName=RegInpADCF1DR12
  Data Store Read7 : DataStoreRead  DataStoreName=RegInpADCF1DR14
  Data Store Read8 : DataStoreRead  DataStoreName=RegInpADCF1DR16
  Data Store Read9 : DataStoreRead  DataStoreName=RegInpADCF1DR18
  Data Type Conversion{,1..11} (12 alike) : DataTypeConversion  OutDataTypeStr=uint32
  Shift Arithmetic{,1..11} (12 alike) : ArithShift  BitShiftNumber=16
  Terminator{1..9} (9 alike) : Terminator
  Unity Scaling Factor1 : Constant  RequirementInfo="{'linktype_rmi_doors' '00016ba8 (/ESG Group/FDD Module Requirements/EA4 Specific/CM012A_FordT3McuCfg)' '#CM012A_184' 'true' 'REQ:  CM012A_184' '' } %GIDa_c79e215a_1c94_4cf9_b554_9d31ad386919"  Value=BATTVLTGSWD1SCAGFAC_ULS_F32  OutDataTypeStr=single
  Unity Scaling Factor{2,4..5,7,9..12,19..21} (11 alike) : Constant  OutDataTypeStr=single
  Unity Scaling Factor3 : Constant  RequirementInfo="{'linktype_rmi_doors' '00016ba8 (/ESG Group/FDD Module Requirements/EA4 Specific/CM012A_FordT3McuCfg)' '#CM012A_179' 'true' 'REQ:  CM012A_179' '' } %GIDa_70a70fc7_f49a_48c6_8c18_ca3e994b4835"  Value=CHRGPMPDIAGSCAGFAC_ULS_F32
  Unity Scaling Factor6 : Constant  RequirementInfo="{'linktype_rmi_doors' '00016ba8 (/ESG Group/FDD Module Requirements/EA4 Specific/CM012A_FordT3McuCfg)' '#CM012A_180' 'true' 'REQ:  CM012A_180' '' } %GIDa_893b80bc_4960_4460_8a5e_9ee1c383990e"  Value=PWRDISCNCTSWTDIAGSCAGFAC_ULS_F32
  Unity Scaling Factor8 : Constant  RequirementInfo="{'linktype_rmi_doors' '00016ba8 (/ESG Group/FDD Module Requirements/EA4 Specific/CM012A_FordT3McuCfg)' '#CM012A_185' 'true' 'REQ:  CM012A_185' '' } %GIDa_ea46589f_3043_4476_970c_fdf6b6000ed0"  Value=BATTVLTGSCAGFAC_ULS_F32  OutDataTypeStr=single
  Adc1ScanGroup3Ref0 : Outport
  EcuT : Outport  Port=2
  ChrgPmpDiag : Outport  Port=3
  PwrDiscnctSwtDiag : Outport  Port=4
  MotAg2Cos : Outport  Port=5
  BattRtnCurrAdc : Outport  Port=6
  MotAg2Sin : Outport  Port=7
  BattVltgSwd1 : Outport  Port=8
  Adc1ScanGroup3Ref1 : Outport  Port=9
  Adc1ScanGroup2Ref0 : Outport  Port=10
  BattVltg : Outport  Port=11
  Adc1ScanGroup2Ref1 : Outport  Port=12
  Adc1SelfDiag0 : Outport  Port=13
  Adc1SelfDiag2 : Outport  Port=14
  Adc1SelfDiag4 : Outport  Port=15
  wires:
  Data Store Read/1 -> Data Type Conversion11/1
  Bitwise Operator/1 -> Convert Adc Results/1
  Unity Scaling Factor4/1 -> Convert Adc Results/2
  Convert Adc Results/1 -> Adc1ScanGroup3Ref0/1
  Shift Arithmetic1/1 -> Convert Adc Results4/1
  Unity Scaling Factor3/1 -> Convert Adc Results3/2
  Bitwise Operator1/1 -> Convert Adc Results3/1
  Unity Scaling Factor2/1 -> Convert Adc Results2/2
  Shift Arithmetic/1 -> Convert Adc Results2/1
  Unity Scaling Factor6/1 -> Convert Adc Results4/2
  Bitwise Operator4/1 -> Convert Adc Results9/1
  Unity Scaling Factor1/1 -> Convert Adc Results8/2
  Shift Arithmetic3/1 -> Convert Adc Results8/1
  Unity Scaling Factor7/1 -> Convert Adc Results7/2
  Unity Scaling Factor5/1 -> Convert Adc Results6/2
  Shift Arithmetic2/1 -> Convert Adc Results6/1
  Bitwise Operator2/1 -> Convert Adc Results5/1
  Unity Scaling Factor9/1 -> Convert Adc Results5/2
  Unity Scaling Factor10/1 -> Convert Adc Results9/2
  Convert Adc Results2/1 -> EcuT/1
  Convert Adc Results3/1 -> ChrgPmpDiag/1
  Convert Adc Results4/1 -> PwrDiscnctSwtDiag/1
  Convert Adc Results5/1 -> MotAg2Cos/1
  Convert Adc Results6/1 -> BattRtnCurrAdc/1
  Convert Adc Results8/1 -> BattVltgSwd1/1
  Convert Adc Results9/1 -> Adc1ScanGroup3Ref1/1
  Convert Adc Results7/1 -> MotAg2Sin/1
  Bitwise Operator3/1 -> Convert Adc Results7/1
  Shift Arithmetic4/1 -> Convert Adc Results10/1
  Unity Scaling Factor11/1 -> Convert Adc Results10/2
  Convert Adc Results10/1 -> Adc1ScanGroup2Ref0/1
  Unity Scaling Factor8/1 -> Convert Adc Results1/2
  Bitwise Operator5/1 -> Convert Adc Results1/1
  Convert Adc Results1/1 -> BattVltg/1
  Shift Arithmetic5/1 -> Convert Adc Results11/1
  Unity Scaling Factor12/1 -> Convert Adc Results11/2
  Convert Adc Results11/1 -> Adc1ScanGroup2Ref1/1
  Unity Scaling Factor21/1 -> Convert Adc Results21/2
  Unity Scaling Factor20/1 -> Convert Adc Results20/2
  Unity Scaling Factor19/1 -> Convert Adc Results19/2
  Shift Arithmetic11/1 -> Convert Adc Results21/1
  Bitwise Operator11/1 -> Convert Adc Results20/1
  Shift Arithmetic10/1 -> Convert Adc Results19/1
  Convert Adc Results21/1 -> Adc1SelfDiag4/1
  Convert Adc Results20/1 -> Adc1SelfDiag2/1
  Convert Adc Results19/1 -> Adc1SelfDiag0/1
  Shift Arithmetic8/1 -> Terminator5/1
  Shift Arithmetic7/1 -> Terminator3/1
  Bitwise Operator8/1 -> Terminator4/1
  Bitwise Operator7/1 -> Terminator6/1
  Bitwise Operator6/1 -> Terminator1/1
  Shift Arithmetic6/1 -> Terminator2/1
  Bitwise Operator9/1 -> Terminator7/1
  Shift Arithmetic9/1 -> Terminator9/1
  Bitwise Operator10/1 -> Terminator8/1
  Data Type Conversion/1 -> Shift Arithmetic11/1, Bitwise Operator11/1
  Data Type Conversion1/1 -> Shift Arithmetic10/1, Bitwise Operator10/1
  Data Type Conversion2/1 -> Bitwise Operator9/1, Shift Arithmetic9/1
  Data Type Conversion3/1 -> Bitwise Operator8/1, Shift Arithmetic8/1
  Data Type Conversion4/1 -> Bitwise Operator7/1, Shift Arithmetic7/1
  Data Type Conversion5/1 -> Bitwise Operator6/1, Shift Arithmetic6/1
  Data Type Conversion6/1 -> Bitwise Operator5/1, Shift Arithmetic5/1
  Data Type Conversion8/1 -> Bitwise Operator3/1, Shift Arithmetic3/1
  Data Type Conversion7/1 -> Bitwise Operator4/1, Shift Arithmetic4/1
  Data Type Conversion9/1 -> Bitwise Operator2/1, Shift Arithmetic2/1
  Data Type Conversion10/1 -> Bitwise Operator1/1, Shift Arithmetic1/1
  Data Type Conversion11/1 -> Bitwise Operator/1, Shift Arithmetic/1
  Data Store Read1/1 -> Data Type Conversion10/1
  Data Store Read2/1 -> Data Type Conversion9/1
  Data Store Read3/1 -> Data Type Conversion8/1
  Data Store Read4/1 -> Data Type Conversion7/1
  Data Store Read5/1 -> Data Type Conversion6/1
  Data Store Read6/1 -> Data Type Conversion5/1
  Data Store Read7/1 -> Data Type Conversion4/1
  Data Store Read8/1 -> Data Type Conversion3/1
  Data Store Read9/1 -> Data Type Conversion2/1
  Data Store Read10/1 -> Data Type Conversion1/1
  Data Store Read11/1 -> Data Type Conversion/1

== system CM012A_FordT3McuCfg/FordT3McuCfg/FordT3McuCfgInit5/CopyRight2 ==

== system CM012A_FordT3McuCfg/FordT3McuCfg/FordT3McuCfgInit5/If Action Subsystem ==
  Action Port : ActionPort  ActionType=then
  Constant : Constant  OutDataTypeStr=uint8
  Constant1 : Constant  Value=MOTAG2MEAS_ECU1OFFS_MOTREV_F32
  CopyRight2 : Subsystem  Description=|  mask(Copyright Information){none=on}
      | Copyright info block.                                               
      |                                                                     
      | Place copyright information at the top of every subsystem in design.
      mask prompts: none "No parameters"
      mask help: Place copyright information at the top of every subsystem in design.
      mask Display:
      | NxtrConf = 'Nexteer Confidential';
      | 
      | sys = bdroot; %handle for the current model ("system")
      | first = get_param(sys,'Created');
      | first = first(end-3:end);  %year is last four digits
      | 
      | last = get_param(sys,'LastModifiedDate');
      | if isempty(last)
      |     last = datestr(now,'yyyy');
      | else
      |     last = last(end-3:end);
      | end
      | 
      | if strcmp(first,last)
      |     fprintf('%s -- Copyright %s Nexteer',NxtrConf,first)
      | else
      |     fprintf('%s -- %s%s- %s Nexteer',NxtrConf,char(169),first,last)
      | end
  Enumerated Constant : simulink/Sources/Enumerated Constant  OutDataTypeStr=Enum: HwAgSnsrTyp1  Value=HwAgSnsrTyp1.HWAGSNSRTYP_A1335  SampleTime=inf
  HwAg1SnsrTyp : Outport
  HwAg1SnsrNr : Outport  Port=2
  MotAg2MeasOffs : Outport  Port=3
  wires:
  Enumerated Constant/1 -> HwAg1SnsrTyp/1
  Constant/1 -> HwAg1SnsrNr/1
  Constant1/1 -> MotAg2MeasOffs/1

== system CM012A_FordT3McuCfg/FordT3McuCfg/FordT3McuCfgInit5/If Action Subsystem3 ==
  Action Port : ActionPort  ActionType=else
  Constant : Constant  Value=0  OutDataTypeStr=uint8
  Constant1 : Constant  Value=MOTAG2MEAS_ECU2OFFS_MOTREV_F32
  CopyRight2 : Subsystem  Description=|  mask(Copyright Information){none=on}
      | Copyright info block.                                               
      |                                                                     
      | Place copyright information at the top of every subsystem in design.
      mask prompts: none "No parameters"
      mask help: Place copyright information at the top of every subsystem in design.
      mask Display:
      | NxtrConf = 'Nexteer Confidential';
      | 
      | sys = bdroot; %handle for the current model ("system")
      | first = get_param(sys,'Created');
      | first = first(end-3:end);  %year is last four digits
      | 
      | last = get_param(sys,'LastModifiedDate');
      | if isempty(last)
      |     last = datestr(now,'yyyy');
      | else
      |     last = last(end-3:end);
      | end
      | 
      | if strcmp(first,last)
      |     fprintf('%s -- Copyright %s Nexteer',NxtrConf,first)
      | else
      |     fprintf('%s -- %s%s- %s Nexteer',NxtrConf,char(169),first,last)
      | end
  Enumerated Constant : simulink/Sources/Enumerated Constant  OutDataTypeStr=Enum: HwAgSnsrTyp1  Value=HwAgSnsrTyp1.HWAGSNSRTYP_NOSNSR  SampleTime=inf
  HwAg1SnsrTyp : Outport
  HwAg1SnsrNr : Outport  Port=2
  MotAg2MeasOffs : Outport  Port=3
  wires:
  Enumerated Constant/1 -> HwAg1SnsrTyp/1
  Constant/1 -> HwAg1SnsrNr/1
  Constant1/1 -> MotAg2MeasOffs/1

== system CM012A_FordT3McuCfg/FordT3McuCfg/FordT3McuCfgPer1/CopyRight2 ==

== system CM012A_FordT3McuCfg/FordT3McuCfg/FordT3McuCfgPer2/CopyRight2 ==

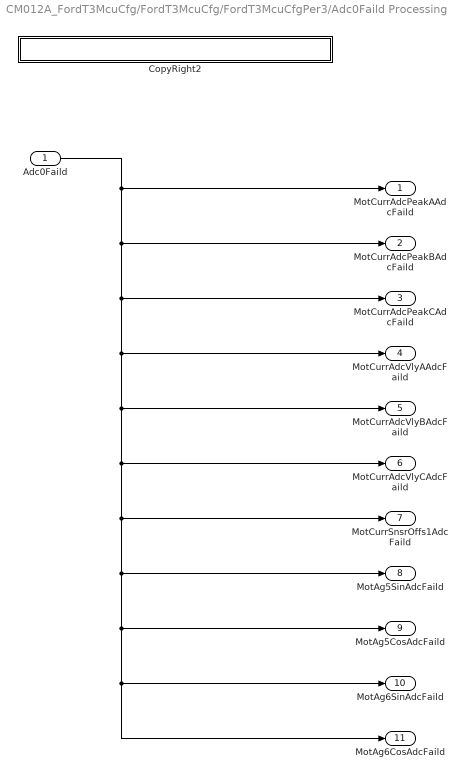
== system CM012A_FordT3McuCfg/FordT3McuCfg/FordT3McuCfgPer3/Adc0Faild Processing ==
  Adc0Faild : Inport
  CopyRight2 : Subsystem  Description=|  mask(Copyright Information){none=on}
      | Copyright info block.                                               
      |                                                                     
      | Place copyright information at the top of every subsystem in design.
      mask prompts: none "No parameters"
      mask help: Place copyright information at the top of every subsystem in design.
      mask Display:
      | NxtrConf = 'Nexteer Confidential';
      | 
      | sys = bdroot; %handle for the current model ("system")
      | first = get_param(sys,'Created');
      | first = first(end-3:end);  %year is last four digits
      | 
      | last = get_param(sys,'LastModifiedDate');
      | if isempty(last)
      |     last = datestr(now,'yyyy');
      | else
      |     last = last(end-3:end);
      | end
      | 
      | if strcmp(first,last)
      |     fprintf('%s -- Copyright %s Nexteer',NxtrConf,first)
      | else
      |     fprintf('%s -- %s%s- %s Nexteer',NxtrConf,char(169),first,last)
      | end
  MotCurrAdcPeakAAdcFaild : Outport
  MotCurrAdcPeakBAdcFaild : Outport  Port=2
  MotCurrAdcPeakCAdcFaild : Outport  Port=3
  MotCurrAdcVlyAAdcFaild : Outport  Port=4
  MotCurrAdcVlyBAdcFaild : Outport  Port=5
  MotCurrAdcVlyCAdcFaild : Outport  Port=6
  MotCurrSnsrOffs1AdcFaild : Outport  Port=7
  MotAg5SinAdcFaild : Outport  Port=8
  MotAg5CosAdcFaild : Outport  Port=9
  MotAg6SinAdcFaild : Outport  Port=10
  MotAg6CosAdcFaild : Outport  Port=11
  wires:
  Adc0Faild/1 -> MotCurrAdcPeakAAdcFaild/1, MotCurrAdcPeakBAdcFaild/1, MotCurrAdcPeakCAdcFaild/1, MotCurrAdcVlyAAdcFaild/1, MotCurrAdcVlyBAdcFaild/1, MotCurrAdcVlyCAdcFaild/1, MotCurrSnsrOffs1AdcFaild/1, MotAg5SinAdcFaild/1, MotAg5CosAdcFaild/1, MotAg6SinAdcFaild/1, MotAg6CosAdcFaild/1

== system CM012A_FordT3McuCfg/FordT3McuCfg/FordT3McuCfgPer3/Adc1Faild Processing ==
  Adc1Faild : Inport
  CopyRight2 : Subsystem  Description=|  mask(Copyright Information){none=on}
      | Copyright info block.                                               
      |                                                                     
      | Place copyright information at the top of every subsystem in design.
      mask prompts: none "No parameters"
      mask help: Place copyright information at the top of every subsystem in design.
      mask Display:
      | NxtrConf = 'Nexteer Confidential';
      | 
      | sys = bdroot; %handle for the current model ("system")
      | first = get_param(sys,'Created');
      | first = first(end-3:end);  %year is last four digits
      | 
      | last = get_param(sys,'LastModifiedDate');
      | if isempty(last)
      |     last = datestr(now,'yyyy');
      | else
      |     last = last(end-3:end);
      | end
      | 
      | if strcmp(first,last)
      |     fprintf('%s -- Copyright %s Nexteer',NxtrConf,first)
      | else
      |     fprintf('%s -- %s%s- %s Nexteer',NxtrConf,char(169),first,last)
      | end
  BattVltgAdcFaild : Outport
  EcuTAdcFaild : Outport  Port=2
  ChrgPmpDiagAdcFaild : Outport  Port=3
  PwrDiscnctSwtDiagAdcFaild : Outport  Port=4
  MotAg2CosAdcFaild : Outport  Port=5
  BattRtnCurrAdcFaild : Outport  Port=6
  MotAg2SinAdcFaild : Outport  Port=7
  BattVltgSwd1AdcFaild : Outport  Port=8
  wires:
  Adc1Faild/1 -> BattVltgSwd1AdcFaild/1, MotAg2SinAdcFaild/1, BattRtnCurrAdcFaild/1, MotAg2CosAdcFaild/1, PwrDiscnctSwtDiagAdcFaild/1, ChrgPmpDiagAdcFaild/1, EcuTAdcFaild/1, BattVltgAdcFaild/1

== system CM012A_FordT3McuCfg/FordT3McuCfg/FordT3McuCfgPer3/CopyRight2 ==

== system CM012A_FordT3McuCfg/FordT3McuCfg/FordT3McuCfgInit1/Register Initialization/CopyRight2 ==

== system CM012A_FordT3McuCfg/FordT3McuCfg/FordT3McuCfgInit2/Register Initialization/CopyRight2 ==

== system CM012A_FordT3McuCfg/FordT3McuCfg/FordT3McuCfgInit3/Process Initial Adc0/CopyRight2 ==

== system CM012A_FordT3McuCfg/FordT3McuCfg/FordT3McuCfgInit3/Wait for ADC Conversion to Complete/CopyRight2 ==

== system CM012A_FordT3McuCfg/FordT3McuCfg/FordT3McuCfgInit3/Wait for ADC Conversion to Complete/GetRefTmr1MicroSec32bit ==
  CopyRight2 : Subsystem  Description=|  mask(Copyright Information){none=on}
      | Copyright info block.                                               
      |                                                                     
      | Place copyright information at the top of every subsystem in design.
      mask prompts: none "No parameters"
      mask help: Place copyright information at the top of every subsystem in design.
      mask Display:
      | NxtrConf = 'Nexteer Confidential';
      | 
      | sys = bdroot; %handle for the current model ("system")
      | first = get_param(sys,'Created');
      | first = first(end-3:end);  %year is last four digits
      | 
      | last = get_param(sys,'LastModifiedDate');
      | if isempty(last)
      |     last = datestr(now,'yyyy');
      | else
      |     last = last(end-3:end);
      | end
      | 
      | if strcmp(first,last)
      |     fprintf('%s -- Copyright %s Nexteer',NxtrConf,first)
      | else
      |     fprintf('%s -- %s%s- %s Nexteer',NxtrConf,char(169),first,last)
      | end
  Ground : Ground
  RefTmr : Outport
  wires:
  Ground/1 -> RefTmr/1
